simulink model "Citation_FlightGear_v2"  (R2026a)
settings: Solver=ode5  StopTime=10  FixedStep=0.01  EnableMultiTasking=on
InitFcn:
  | run('initcit.m')
  | run('id_init.m')
values from neighbouring files (symbols this model uses):
  beta_ref_max = 5*pi/180    (= 0.0872664625997)    [id_init.m]
  K_beta = 2    [id_init.m]
  K_da_to_p = p_ref_max/0.65    (= 0.537024385229)    [id_init.m]
  K_de_to_q = q_ref_max/0.35    (= 0.49866550057)    [id_init.m]
  K_dr_to_beta = beta_ref_max/0.38    (= 0.229648585789)    [id_init.m]
  Kaw_p = 1/Taw_p    (= 2)    [id_init.m]
  Kaw_q = 1/Taw_q    (= 2)    [id_init.m]
  Kaw_r = 1/Taw_r    (= 2)    [id_init.m]
  Ki_p = 5.0    (= 5)    [id_init.m]
  Ki_p_classical = -0.5    [id_init.m]
  Ki_q = 5.0    (= 5)    [id_init.m]
  Ki_q_classical = -0.1    [id_init.m]
  Ki_r = 5.0    (= 5)    [id_init.m]
  Ki_r_classical = -0.1    [id_init.m]
  Kp_p = 4.5    [id_init.m]
  Kp_p_classical = -1    [id_init.m]
  Kp_q = 4.5    [id_init.m]
  Kp_q_classical = -2    [id_init.m]
  Kp_r = 4.5    [id_init.m]
  Kp_r_classical = -2    [id_init.m]
  p_ref_max = 20*pi/180    (= 0.349065850399)    [id_init.m]
  PL0 = 10000*eye(6)    [id_init.m]
  PM0 = 10000*eye(4)    [id_init.m]
  PN0 = 10000*eye(6)    [id_init.m]
  PX0 = 10000*eye(5)    [id_init.m]
  PY0 = 10000*eye(6)    [id_init.m]
  PZ0 = 10000*eye(4)    [id_init.m]
  q_ref_max = 10*pi/180    (= 0.174532925199)    [id_init.m]
  r_ref_max = 10*pi/180    (= 0.174532925199)    [id_init.m]
  tau_cmd = 0.5    [id_init.m]
  thetaL0 = [       7.0957952465296537e-06 ... (first row only)    [id_init.m]
  thetaM0 = [       1.2280209971618383e-02 ... (first row only)    [id_init.m]
  thetaN0 = [      -4.9609095125384690e-06 ... (first row only)    [id_init.m]
  thetaX0 = zeros(5,1)    [id_init.m]
  thetaY0 = zeros(6,1)    [id_init.m]
  thetaZ0 = zeros(4,1)    [id_init.m]
  TL = 7.0875e-06    [id_init.m]
  TM = 3.2564e-06    [id_init.m]
  TN = 5.4692e-07    [id_init.m]
  TX = 2.2784e-06    [id_init.m]
  TY = 8.0633e-07    [id_init.m]
  TZ = 2.8004e-05    [id_init.m]
  Vw915 = 0    [initcit.m]
  winddir = -27*(pi/180)    (= -0.471238898038)    [initcit.m]
  x0 = []    [cessnac550_3d_sfnc.m]
undefined symbols (not defined in the file or in its folder): chord, cv1, cv2, cv3, cv4, deltagmax1, deltagmax2, deltagmax3, deltagmax4, Deng, ealphag, ealphas, g0, hDME, hGS, kt1, kt2, kt3, lh, massinit, matbuaf, matdaf, matdam, matdbbf, matdeaf, matdgaf, matdqaf, matduaf, matdwaw, matedhr, mateif, matelhr, matemhr, matemv1, matemv2, matemve, matetam, mateuaf, matfaaf, matfaxl, matff, matibaf, matibb, matibmh, matipaf, matipmh, matiraf, matiuaf, matiwaf, matlaf, matlam, matleaf, matleam, matlgaf, matlqaf, matluaf, matmaaf, matmaam, matmaf, matmam ... (+78)
libraries: simulink x13, aerolibfltsims x3, aerolibconvert2 x2, aerolibobsolete x1, aerolibanimutils x1
(part 1 of 5)
settings Model: ExtModeTrigMode=oneshot  ExtModeArmWhenConnect=off  Creator=laurensvaneykeren  LastModifiedBy=eltjo
settings DataIOCC: SignalLoggingSaveFormat=ModelDataLogs  SignalLoggingName=sigsOut
settings OptimizationCC: BooleanDataType=off
settings DebuggingCC: SaveWithParameterizedLinksMsg=none  UnderspecifiedInitializationDetection=Classic  SignalResolutionControl=TryResolveAllWithWarning  MultiTaskDSMMsg=warning  MultiTaskCondExecSysMsg=none
settings HardwareCC: ProdHWDeviceType=32-bit Generic  TargetUnknown=on
settings RTWCC: SystemTargetFile=grt_malloc.tlc  GenCodeOnly=on  TemplateMakefile=grt_malloc_default_tmf
settings GRTTargetCC: UseMalloc=on  CombineOutputUpdateFcns=off  GRTInterface=on

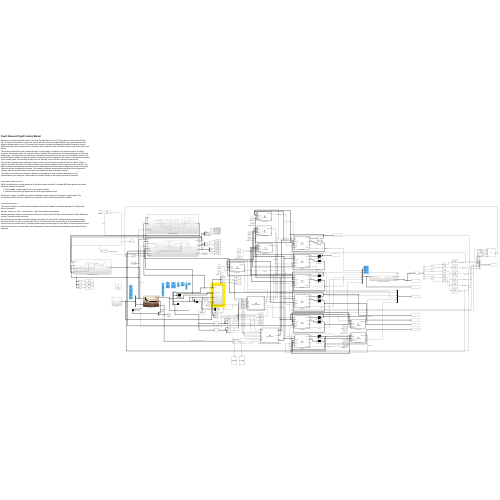
[thumbnail: Simulink's stored preview of the top-level diagram]
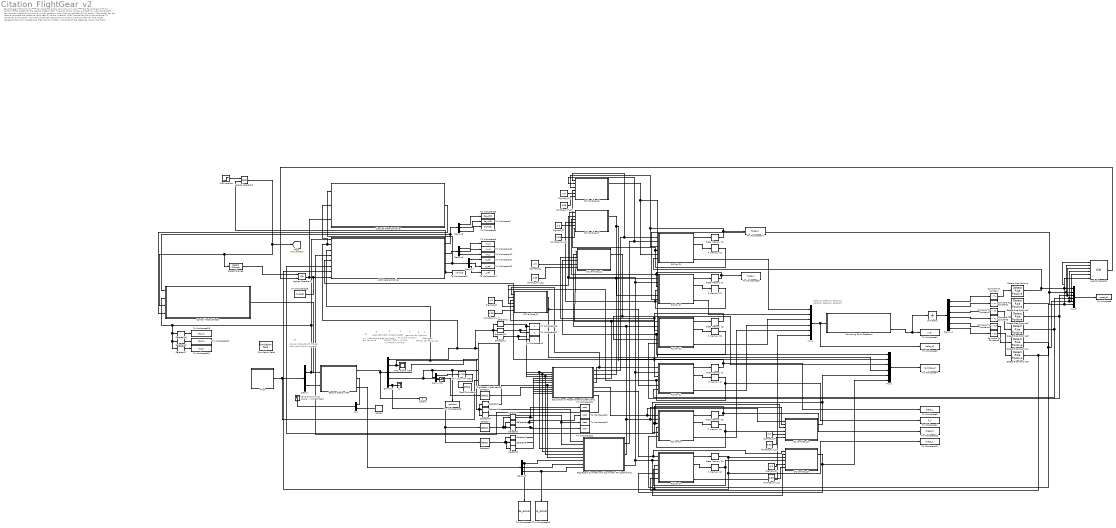
== system Citation_FlightGear_v2 ==
  note: Fault-Tolerant Flight Control Model
      | Welcome to the main Simulink model of the Fault-Tolerant Flight Control (FTFC) system for the Cessna Citation 500. The goal of this model is to test how well the aircraft can maintain stable flight during normal operation and when an actuator failure occurs. The model can be used to compare the Adaptive Nonlinear Dynamic Inversion (ANDI) controller with a conventional PI controller, and to study how both controllers respond to an aileron hard-over failure.
      | The model represents the main closed-loop flight control system. It consists of the reference inputs, the flight controller, the actuator model, the nonlinear Cessna Citation 500 aircraft model, the feedback signals, and the fault-related logic. The reference inputs specify the desired aircraft response and are sent to the selected controller. The controller then calculates the required actuator commands, which are passed to the actuator subsystem and applied to the aircraft model. The resulting aircraft motion is fed back to the controller, closing the control loop.
      | The actuator subsystem also contains the failure model used to introduce the aileron hard-over failure. When a failure is activated, the effect of the failed actuator can be studied together with the response of the controller. The ANDI controller uses feedback information and the estimated control effectiveness to adjust the control commands when the actuator configuration changes. This makes it possible to compare the nominal and failure cases and evaluate how well the fault-tolerant controller can maintain the desired aircraft behaviour.
      | The model can therefore be operated in different configurations to study controller performance, fault accommodation and tolerance, and the effect of actuator failures on the closed-loop aircraft dynamics.
      |
      | Switching Between ANDI and PI Control
      | ANDI is enabled during normal operation of the fault-tolerant controller. To disable ANDI and operate the aircraft using the classical PI controller:
      | Set the ANDI enable signal to 0 for the entire simulation.
      | Disconnect the valid_B signal from the AND logical operator block.
      | With these changes, the ANDI control path is disabled and the classical PI controller is used instead. This configuration can be used as a baseline for comparison with the fault-tolerant ANDI controller.
      |
      | Activating the Actuator Failure
      | The model contains an actuator failure mechanism that can be enabled or disabled manually. To configure the failure, navigate to:
      | Cessna Citation 500 → Actuators → Failure Mode Activation
      | Enabling Failure Mode Activation introduces an aileron hard-over failure into the aircraft model. Disabling it restores nominal actuator behaviour.
      | By combining the controller and failure settings, the model can be used to investigate several important cases, including nominal PI control, nominal ANDI control, PI control during an actuator failure, and fault-tolerant ANDI control during an actuator failure. Comparing these cases provides insight into the ability of the fault-tolerant control architecture to detect, accommodate, and compensate for actuator failures while maintaining the desired aircraft response.
  note: de
      | da
      | dr
      | dte
      | dta
      | dtr
      | df
      | gear
      | pla1
      | pla2
      | turb 8x
      | terr elev
  note: p
      | q
      | r
      | vtas
      | alpha
      | beta
      | phi
      | theta
      | psi
      | he
      | xe
      | ye
  note: pdot
      | qdot
      | rdot
      | VTASdot
      | hedot
  note: hradio
      | Mach
      | u_wind_e
      | v_wind_e
      | w_wind_e
  note: anxb
      | anyb
      | anzb
      | n
  note: gamma
      | chi
      | Vground
  note: flaps
      | gear
  note: FFl
      | N1l
      | N2l
      | FFr
      | N1r
      | N2r
  note: 12
  note: 5
  note: 5
  note: 4
  note: 3
  note: 6
  note: 2
  note: 19
  note: delta_CX
      | delta_CY
      | delta_CZ
      | delta_Cl
      | delta_Cm
      | delta_Cn
  2 : Terminator
  3 : Terminator
  ANDI Rate Controller : Subsystem
  ANDI enable : Step  Time=0  InitialValue=1  SampleTime=0
  Alt < 10 m => Stop : Fcn  Expr=u<10
  CIC lambda_CX : MATLAB Function  TreatAsAtomicUnit=on
  CIC lambda_CY : MATLAB Function  TreatAsAtomicUnit=on
  CIC lambda_CZ : MATLAB Function  TreatAsAtomicUnit=on
  CIC lambda_Cl : MATLAB Function  TreatAsAtomicUnit=on
  CIC lambda_Cm : MATLAB Function  TreatAsAtomicUnit=on
  CIC lambda_Cn : MATLAB Function  TreatAsAtomicUnit=on
  Calculation of Force/Moments Coefficients : MATLAB Function  TreatAsAtomicUnit=on
  Cessna Citation 500 : Subsystem  mask(Citation Aircraft Model){trimdatafile=}
      mask prompts: trimdatafile "Trim Condition"
      mask init:
      | initcit;
      mask Display:
      | image(imread('Citation.jpg'))
      | port_label('input', 1, 'Inputs')
      | port_label('input', 2, 'Environment')
      | port_label('output', 1, 'Outputs')
      | port_label('output', 2, 'Trim inputs')
  Classical Rate Controller : Subsystem
  Compare To Constant : simulink/Logic and Bit Operations/Compare To Constant  relop=>  const=TX  OutDataTypeStr=boolean
  Compare To Constant1 : simulink/Logic and Bit Operations/Compare To Constant  relop=>  const=TY  OutDataTypeStr=boolean
  Compare To Constant2 : simulink/Logic and Bit Operations/Compare To Constant  relop=>  const=TZ  OutDataTypeStr=boolean
  Compare To Constant3 : simulink/Logic and Bit Operations/Compare To Constant  relop=>  const=TL  OutDataTypeStr=boolean
  Compare To Constant4 : simulink/Logic and Bit Operations/Compare To Constant  relop=>  const=TM  OutDataTypeStr=boolean
  Compare To Constant5 : simulink/Logic and Bit Operations/Compare To Constant  relop=>  const=TN  OutDataTypeStr=boolean
  Control Mode Selector : Subsystem
  Demux : Demux  Outputs=[10 9]
      settings: DisplayOption=none
  Demux1 : Demux  Outputs=[3 3 3 3 25]
      settings: DisplayOption=none
  Demux2 : Demux  Outputs=[1 2]
  Demux{3,5..7} (4 alike) : Demux  Outputs=3
  Demux4 : Demux  Outputs=6
  Detect Change : simulink/Logic and Bit Operations/Detect Change  vinit=0  OutDataTypeStr=boolean
  Detect Rise Positive{,1..5} (6 alike) : simulink/Logic and Bit Operations/Detect Rise Positive  vinit=0  OutDataTypeStr=boolean
  FlightGear Visualisation : Subsystem
  Logical Operator : Logic  Operator=OR  Inputs=6  AllPortsSameDT=off  OutDataTypeStr=boolean
  Logical Operator1 : Logic  Operator=OR  AllPortsSameDT=off  OutDataTypeStr=boolean
  Logical Operator2 : Logic  AllPortsSameDT=off  OutDataTypeStr=boolean
  Monitoring Fault Detection : Subsystem
  Mux : Mux  Inputs=2
  Mux1 : Mux  Inputs=6
  Mux2 : Mux  Inputs=6
  Mux3 : Mux  Inputs=6
  P memory CX : Memory  InitialCondition=PX0
  P memory CY : Memory  InitialCondition=PY0
  P memory CZ : Memory  InitialCondition=PZ0
  P memory Cl : Memory  InitialCondition=PL0
  P memory Cm : Memory  InitialCondition=PM0
  P memory Cn : Memory  InitialCondition=PN0
  Pilot : Subsystem
  RLS for CL : MATLAB Function  TreatAsAtomicUnit=on
  RLS for CX : MATLAB Function  TreatAsAtomicUnit=on
  RLS for CY : MATLAB Function  TreatAsAtomicUnit=on
  RLS for CZ : MATLAB Function  TreatAsAtomicUnit=on
  RLS for Cm : MATLAB Function  TreatAsAtomicUnit=on
  RLS for Cn : MATLAB Function  TreatAsAtomicUnit=on
  Regressors Symmetr. and Asymmetr. F/M Coefficients : MATLAB Function  TreatAsAtomicUnit=on
  Selector : Selector  InputPortWidth=25  IndexOptions=Index vector (dialog)  Indices=[1 2 3]  OutputSizes=1
  Selector1 : Selector  InputPortWidth=3  IndexOptions=Index vector (dialog)  Indices=1  OutputSizes=1
  Selector{5,8,10,13} (4 alike) : Selector  InputPortWidth=3  IndexOptions=Index vector (dialog)  Indices=[2]  OutputSizes=1
  Selector{6,9,11,14} (4 alike) : Selector  InputPortWidth=3  IndexOptions=Index vector (dialog)  Indices=[3]  OutputSizes=1
  Selector{3..4,7,12} (4 alike) : Selector  InputPortWidth=3  IndexOptions=Index vector (dialog)  Indices=[1]  OutputSizes=1
  Selector15 : Selector  InputPortWidth=10  IndexOptions=Index vector (dialog)  Indices=[1]  OutputSizes=1
  Selector16 : Selector  InputPortWidth=10  IndexOptions=Index vector (dialog)  Indices=[2]  OutputSizes=1
  Selector17 : Selector  InputPortWidth=10  IndexOptions=Index vector (dialog)  Indices=[3]  OutputSizes=1
  Selector2 : Selector  InputPortWidth=25  IndexOptions=Index vector (dialog)  Indices=[11 12 13]  OutputSizes=1
  Sigma0_CX : Constant  Value=0.5
  Sigma0_CY : Constant  Value=0.5
  Sigma0_CZ : Constant  Value=0.5
  Sigma0_Cl : Constant  Value=0.5
  Sigma0_Cm : Constant  Value=0.5
  Sigma0_Cn : Constant  Value=0.5
  Simulation Pace : aerolibanimutils/Simulation Pace  SimulationPace=1  SleepMode=MATLAB Thread  OutputPaceError=off  SampleTime=-1
      settings: AttributesFormatString=%<SimulationPace> sec/sec
  Stop Simulation : Stop
  To Workspace : ToWorkspace  VariableName=reset_all  SaveFormat=Timeseries  SampleTime=-1
  To Workspace1 : ToWorkspace  VariableName=P_L  SaveFormat=Timeseries  SampleTime=-1
  To Workspace10 : ToWorkspace  VariableName=nu_q  SaveFormat=Timeseries  SampleTime=-1
  To Workspace11 : ToWorkspace  VariableName=p_ref  SaveFormat=Timeseries  SampleTime=-1
  To Workspace12 : ToWorkspace  VariableName=nu_r  SaveFormat=Timeseries  SampleTime=-1
  To Workspace13 : ToWorkspace  VariableName=q_ref  SaveFormat=Timeseries  SampleTime=-1
  To Workspace14 : ToWorkspace  VariableName=r_ref  SaveFormat=Timeseries  SampleTime=-1
  To Workspace15 : ToWorkspace  VariableName=valid_B  SaveFormat=Timeseries  SampleTime=-1
  To Workspace16 : ToWorkspace  VariableName=p  SaveFormat=Timeseries  SampleTime=-1
  To Workspace17 : ToWorkspace  VariableName=q  SaveFormat=Timeseries  SampleTime=-1
  To Workspace18 : ToWorkspace  VariableName=r  SaveFormat=Timeseries  SampleTime=-1
  To Workspace19 : ToWorkspace  VariableName=beta  SaveFormat=Timeseries  SampleTime=-1
  To Workspace2 : ToWorkspace  VariableName=Jvar  SaveFormat=Timeseries  SampleTime=-1
  To Workspace20 : ToWorkspace  VariableName=qdot  SaveFormat=Timeseries  SampleTime=-1
  To Workspace21 : ToWorkspace  VariableName=pdot  SaveFormat=Timeseries  SampleTime=-1
  To Workspace22 : ToWorkspace  VariableName=rdot  SaveFormat=Timeseries  SampleTime=-1
  To Workspace23 : ToWorkspace  VariableName=theta_M  SaveFormat=Timeseries  SampleTime=-1
  To Workspace24 : ToWorkspace  VariableName=theta_N  SaveFormat=Timeseries  SampleTime=-1
  To Workspace25 : ToWorkspace  VariableName=PI_reset  SaveFormat=Timeseries  SampleTime=-1
  To Workspace26 : ToWorkspace  VariableName=theta_Y  SaveFormat=Timeseries  SampleTime=-1
  To Workspace27 : ToWorkspace  VariableName=theta_X  SaveFormat=Timeseries  SampleTime=-1
  To Workspace28 : ToWorkspace  VariableName=position  SaveFormat=Timeseries  SampleTime=-1
  To Workspace29 : ToWorkspace  VariableName=de_joy  SaveFormat=Timeseries  SampleTime=-1
  To Workspace3 : ToWorkspace  VariableName=delta_all  SaveFormat=Timeseries  SampleTime=-1
  To Workspace30 : ToWorkspace  VariableName=da_joy  SaveFormat=Timeseries  SampleTime=-1
  To Workspace31 : ToWorkspace  VariableName=dr_joy  SaveFormat=Timeseries  SampleTime=-1
  To Workspace32 : ToWorkspace  VariableName=de_actual  SaveFormat=Timeseries  SampleTime=-1
  To Workspace33 : ToWorkspace  VariableName=dr_actual  SaveFormat=Timeseries  SampleTime=-1
  To Workspace4 : ToWorkspace  VariableName=lambda_all  SaveFormat=Timeseries  SampleTime=-1
  To Workspace5 : ToWorkspace  VariableName=de_ANDI  SaveFormat=Timeseries  SampleTime=-1
  To Workspace6 : ToWorkspace  VariableName=dr_ANDI  SaveFormat=Timeseries  SampleTime=-1
  To Workspace7 : ToWorkspace  VariableName=da_ANDI  SaveFormat=Timeseries  SampleTime=-1
  To Workspace8 : ToWorkspace  VariableName=theta_L  SaveFormat=Timeseries  SampleTime=-1
  To Workspace9 : ToWorkspace  VariableName=nu_p  SaveFormat=Timeseries  SampleTime=-1
  Unit Delay : UnitDelay  SampleTime=0.01
  Using this as input would result in trimmed flight : Terminator
  "VTAS, alpha, beta" : Scope
      settings: ActiveDisplayYMinimum=-192.0765592563377  ActiveDisplayYMaximum=190.51852643229006  DataLoggingVariableName=ScopeData7
  lambda_min_CX : Constant  Value=0.95
  lambda_min_CY : Constant  Value=0.95
  lambda_min_CZ : Constant  Value=0.95
  lambda_min_Cl : Constant  Value=0.95
  lambda_min_Cm : Constant  Value=0.95
  lambda_min_Cn : Constant  Value=0.95
  theta Memory CX : Memory  InitialCondition=thetaX0
  theta Memory CY : Memory  InitialCondition=thetaY0
  theta Memory CZ : Memory  InitialCondition=thetaZ0
  theta Memory Cl : Memory  InitialCondition=thetaL0
  theta Memory Cm : Memory  InitialCondition=thetaM0
  theta Memory Cn : Memory  InitialCondition=thetaN0
  zeroes : Constant  Value=[0 0 0 0 0 0 0 0 0]
  Output : Outport
  tag scope: ANDI_ENABLE=global
  wires:
  Demux/1 -> Selector17/1, Selector16/1, Selector15/1, Control Mode Selector/2(pilot_u), ANDI Rate Controller/1(pilot_u)
  Cessna Citation 500/1(output) -> Demux1/1, Output/1
  Demux/2 -> Cessna Citation 500/2(Environment)
  Cessna Citation 500/2(Trimmed input) -> Mux/1  "Input values in trim condition"
  zeroes/1 -> Mux/2
  Mux/1 -> Using this as input would result in trimmed flight/1
  Demux1/1 -> Classical Rate Controller/2(pqr), ANDI Rate Controller/2(pqr), Selector11/1, Selector12/1, Selector10/1, FlightGear Visualisation/1("[p,q,r]")  "p,q,r"
  Demux1/2 -> ANDI Rate Controller/3("VTAS, alpha, beta"), Selector14/1, Selector3/1, Selector13/1, "VTAS, alpha, beta"/1
  Alt < 10 m => Stop/1 -> Stop Simulation/1
  Demux1/5 -> Selector2/1, Selector/1, 2/1
  Demux1/4 -> Selector1/1, Demux2/1, To Workspace28/1, FlightGear Visualisation/3("[he, xe, ye]")
  Demux2/1 -> Alt < 10 m => Stop/1
  Pilot/1(Input) -> FlightGear Visualisation/4(u), Demux/1
  Demux2/2 -> 3/1
  Demux1/3 -> FlightGear Visualisation/2(" [phi, theta, psi]")  "phi,theta,psi"
  Cessna Citation 500/3(Outport SysID Deflections) -> Demux3/1  "de_healthy, da_healthy, dr_healthy"
  Selector1/1 -> Calculation of Force/Moments Coefficients/8(h)  "he"
  Selector3/1 -> Regressors Symmetr. and Asymmetr. F/M Coefficients/6(V), Calculation of Force/Moments Coefficients/7(V)  "VTAS"
  Selector/1 -> Selector4/1, Selector5/1, Selector6/1
  Selector4/1 -> To Workspace21/1, Calculation of Force/Moments Coefficients/4(pdot)  "pdot"
  Selector5/1 -> To Workspace20/1, Calculation of Force/Moments Coefficients/5(qdot)  "qdot"
  Selector6/1 -> To Workspace22/1, Calculation of Force/Moments Coefficients/6(rdot)  "rdot"
  Selector7/1 -> Calculation of Force/Moments Coefficients/9(anxb)  "anxb"
  Selector9/1 -> Calculation of Force/Moments Coefficients/11(anzb)  "anzb"
  Selector8/1 -> Calculation of Force/Moments Coefficients/10(anyb)  "anyb"
  Selector2/1 -> Selector9/1, Selector8/1, Selector7/1
  Selector12/1 -> To Workspace16/1, Regressors Symmetr. and Asymmetr. F/M Coefficients/3(p), Calculation of Force/Moments Coefficients/1(p)  "p"
  Selector10/1 -> To Workspace17/1, Regressors Symmetr. and Asymmetr. F/M Coefficients/4(q), Calculation of Force/Moments Coefficients/2(q)  "q"
  Selector11/1 -> To Workspace18/1, Regressors Symmetr. and Asymmetr. F/M Coefficients/5(r), Calculation of Force/Moments Coefficients/3(r)  "r"
  Selector13/1 -> Regressors Symmetr. and Asymmetr. F/M Coefficients/1(alpha)  "alpha"
  Selector14/1 -> Regressors Symmetr. and Asymmetr. F/M Coefficients/2(beta), To Workspace19/1  "beta"
  Demux3/1 -> Regressors Symmetr. and Asymmetr. F/M Coefficients/7(de), To Workspace32/1  "de_healthy"
  Demux3/2 -> Regressors Symmetr. and Asymmetr. F/M Coefficients/8(da)  "da_healthy"
  Demux3/3 -> Regressors Symmetr. and Asymmetr. F/M Coefficients/9(dr), To Workspace33/1  "dr_healthy"
  Regressors Symmetr. and Asymmetr. F/M Coefficients/3(phiLat) -> CIC lambda_Cn/2(phi), RLS for Cn/2(phi), RLS for CL/2(phi), RLS for CY/2(phi), CIC lambda_Cl/2(phi), CIC lambda_CY/2(phi)
  RLS for Cn/1(theta_new) -> theta Memory Cn/1
  theta Memory Cn/1 -> To Workspace24/1, ANDI Rate Controller/7(thetaN), RLS for Cn/3(theta_old), CIC lambda_Cn/3(theta_old)
  RLS for Cn/2(P_new) -> P memory Cn/1
  P memory Cn/1 -> RLS for Cn/4(P_old), CIC lambda_Cn/4(P_old)
  Calculation of Force/Moments Coefficients/1(CX) -> CIC lambda_CX/1(z), RLS for CX/1(z)
  P memory CX/1 -> CIC lambda_CX/4(P_old), RLS for CX/4(P_old)
  theta Memory CX/1 -> CIC lambda_CX/3(theta_old), RLS for CX/3(theta_old), To Workspace27/1
  RLS for CX/2(P_new) -> P memory CX/1
  RLS for CX/1(theta_new) -> theta Memory CX/1
  Regressors Symmetr. and Asymmetr. F/M Coefficients/1(phiX) -> CIC lambda_CX/2(phi), RLS for CX/2(phi)
  P memory CY/1 -> CIC lambda_CY/4(P_old), RLS for CY/4(P_old)
  theta Memory CY/1 -> CIC lambda_CY/3(theta_old), RLS for CY/3(theta_old), To Workspace26/1
  RLS for CY/2(P_new) -> P memory CY/1
  RLS for CY/1(theta_new) -> theta Memory CY/1
  Calculation of Force/Moments Coefficients/2(CY) -> RLS for CY/1(z), CIC lambda_CY/1(z)
  P memory CZ/1 -> RLS for CZ/4(P_old), CIC lambda_CZ/4(P_old)
  theta Memory CZ/1 -> CIC lambda_CZ/3(theta_old), RLS for CZ/3(theta_old)
  CIC lambda_CZ/1(lambda_ad) -> RLS for CZ/5(lambda), Mux2/3  "lambda_CZ"
  RLS for CZ/2(P_new) -> P memory CZ/1
  RLS for CZ/1(theta_new) -> theta Memory CZ/1
  Calculation of Force/Moments Coefficients/3(CZ) -> RLS for CZ/1(z), CIC lambda_CZ/1(z)
  Regressors Symmetr. and Asymmetr. F/M Coefficients/2(phiZM) -> CIC lambda_Cm/2(phi), RLS for Cm/2(phi), RLS for CZ/2(phi), CIC lambda_CZ/2(phi)
  P memory Cl/1 -> To Workspace1/1, CIC lambda_Cl/4(P_old), RLS for CL/4(P_old)
  theta Memory Cl/1 -> To Workspace8/1, ANDI Rate Controller/5(thetaL), RLS for CL/3(theta_old), CIC lambda_Cl/3(theta_old)
  CIC lambda_Cl/1(lambda_ad) -> Mux2/4, RLS for CL/5(lambda)  "lambda_Cl"
  RLS for CL/2(P_new) -> P memory Cl/1
  RLS for CL/1(theta_new) -> theta Memory Cl/1
  P memory Cm/1 -> RLS for Cm/4(P_old), CIC lambda_Cm/4(P_old)
  theta Memory Cm/1 -> To Workspace23/1, ANDI Rate Controller/6(thetaM), CIC lambda_Cm/3(theta_old), RLS for Cm/3(theta_old)
  RLS for Cm/2(P_new) -> P memory Cm/1
  RLS for Cm/1(theta_new) -> theta Memory Cm/1
  Calculation of Force/Moments Coefficients/4(Cl) -> CIC lambda_Cl/1(z), RLS for CL/1(z)
  Calculation of Force/Moments Coefficients/5(Cm) -> CIC lambda_Cm/1(z), RLS for Cm/1(z)
  Calculation of Force/Moments Coefficients/6(Cn) -> CIC lambda_Cn/1(z), RLS for Cn/1(z)
  RLS for CX/4(innovation) -> Mux1/1  "delta_CX"
  RLS for CY/4(innovation) -> Mux1/2  "delta_CY"
  RLS for CZ/4(innovation) -> Mux1/3  "delta_CZ"
  RLS for CL/4(innovation) -> Mux1/4  "delta_Cl"
  RLS for Cm/4(innovation) -> Mux1/5  "delta_Cm"
  RLS for Cn/4(innovation) -> Mux1/6  "delta_Cn"
  Mux1/1 -> To Workspace3/1, Monitoring Fault Detection/1(innovations)
  Sigma0_CX/1 -> CIC lambda_CX/5(Sigma0)
  lambda_min_CX/1 -> CIC lambda_CX/6(lambda_min)
  CIC lambda_CX/1(lambda_ad) -> Mux2/1, RLS for CX/5(lambda)  "lambda_CX"
  Sigma0_CY/1 -> CIC lambda_CY/5(Sigma0)
  lambda_min_CY/1 -> CIC lambda_CY/6(lambda_min)
  CIC lambda_CY/1(lambda_ad) -> Mux2/2, RLS for CY/5(lambda)  "lambda_CY"
  Sigma0_CZ/1 -> CIC lambda_CZ/5(Sigma0)
  lambda_min_CZ/1 -> CIC lambda_CZ/6(lambda_min)
  Sigma0_Cl/1 -> CIC lambda_Cl/5(Sigma0)
  lambda_min_Cl/1 -> CIC lambda_Cl/6(lambda_min)
  Sigma0_Cm/1 -> CIC lambda_Cm/5(Sigma0)
  lambda_min_Cm/1 -> CIC lambda_Cm/6(lambda_min)
  CIC lambda_Cm/1(lambda_ad) -> Mux2/5, RLS for Cm/5(lambda)  "lambda_Cm"
  Sigma0_Cn/1 -> CIC lambda_Cn/5(Sigma0)
  lambda_min_Cn/1 -> CIC lambda_Cn/6(lambda_min)
  CIC lambda_Cn/1(lambda_ad) -> Mux2/6, RLS for Cn/5(lambda)  "lambda_Cn"
  Monitoring Fault Detection/3(VARIANCE) -> Unit Delay/1, To Workspace2/1  "Variance"
  Mux2/1 -> To Workspace4/1
  Demux4/1 -> Compare To Constant/1  "Jvar_X"
  Demux4/2 -> Compare To Constant1/1  "Jvar_Y"
  Demux4/3 -> Compare To Constant2/1  "Jvar_Z"
  Demux4/4 -> Compare To Constant3/1  "Jvar_L"
  Demux4/5 -> Compare To Constant4/1  "Jvar_M"
  Demux4/6 -> Compare To Constant5/1  "Jvar_N"
  Compare To Constant/1 -> Detect Rise Positive/1
  Compare To Constant1/1 -> Detect Rise Positive1/1
  Compare To Constant2/1 -> Detect Rise Positive2/1
  Compare To Constant3/1 -> Detect Rise Positive3/1
  Compare To Constant5/1 -> Detect Rise Positive5/1
  Compare To Constant4/1 -> Detect Rise Positive4/1
  Detect Rise Positive/1 -> RLS for CX/6(reset), Logical Operator/1, Mux3/1  "reset_CX"
  Detect Rise Positive1/1 -> Logical Operator/2, Mux3/2, RLS for CY/6(reset)  "reset_CY"
  Detect Rise Positive2/1 -> RLS for CZ/6(reset), Logical Operator/3, Mux3/3  "reset_CZ"
  Detect Rise Positive3/1 -> RLS for CL/6(reset), Logical Operator/4, Mux3/4  "reset_CL"
  Detect Rise Positive4/1 -> Logical Operator/5, Mux3/5, RLS for Cm/6(reset)  "reset_CM"
  Detect Rise Positive5/1 -> RLS for Cn/6(reset), Mux3/6, Logical Operator/6  "reset_CN"
  Mux3/1 -> To Workspace/1
  Unit Delay/1 -> Demux4/1
  Calculation of Force/Moments Coefficients/7(rho) -> ANDI Rate Controller/4(rho)
  ANDI enable/1 -> Logical Operator2/1
  ANDI Rate Controller/1(u_ANDI) -> Demux5/1, Control Mode Selector/1(u_ANDI)
  Control Mode Selector/1(aircraft_u) -> Cessna Citation 500/1(Inputs)  "aircraft_u"
  Logical Operator/1 -> Logical Operator1/2  "model_reset"
  Detect Change/1 -> Logical Operator1/1  "mode_change"
  Logical Operator1/1 -> Classical Rate Controller/3(PI_reset), To Workspace25/1, ANDI Rate Controller/8(PI_reset)  "PI_reset"
  Demux5/1 -> To Workspace5/1  "de_ANDI"
  Demux5/2 -> To Workspace7/1  "da_ANDI"
  Demux5/3 -> To Workspace6/1  "dr_ANDI"
  ANDI Rate Controller/2(nu) -> Demux6/1
  Demux6/1 -> To Workspace9/1  "nu_p"
  Demux6/2 -> To Workspace10/1  "nu_q"
  Demux6/3 -> To Workspace12/1  "nu_r"
  ANDI Rate Controller/3(refs) -> Classical Rate Controller/1(refs), Demux7/1
  Demux7/1 -> To Workspace11/1  "p_ref"
  Demux7/2 -> To Workspace13/1  "q_ref"
  Demux7/3 -> To Workspace14/1  "r_ref"
  ANDI Rate Controller/4(valid_B) -> To Workspace15/1, Logical Operator2/2  "valid_B"
  Classical Rate Controller/1(u_classical) -> Control Mode Selector/4(u_classical)
  Selector15/1 -> To Workspace29/1
  Selector16/1 -> To Workspace30/1
  Selector17/1 -> To Workspace31/1
  Logical Operator2/1 -> Detect Change/1, Control Mode Selector/3(ANDI_enable), [ANDI_ENABLE]

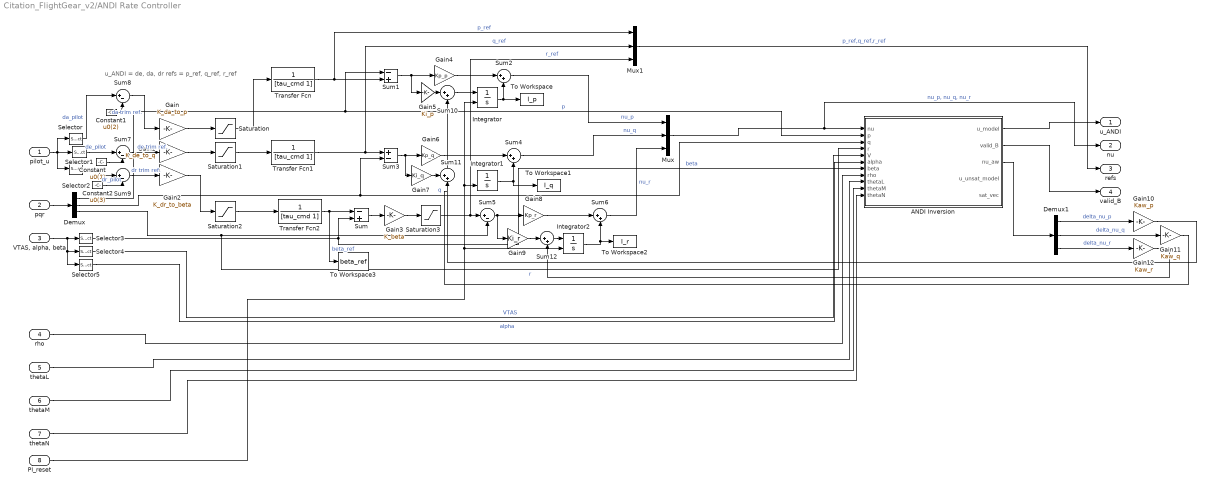
== system Citation_FlightGear_v2/ANDI Rate Controller ==
  note: u_ANDI = de, da, dr
      | refs = p_ref, q_ref, r_ref
  pilot_u : Inport
  pqr : Inport  Port=2
  "VTAS, alpha, beta" : Inport  Port=3
  rho : Inport  Port=4
  thetaL : Inport  Port=5
  thetaM : Inport  Port=6
  thetaN : Inport  Port=7
  PI_reset : Inport  Port=8
  ANDI Inversion : MATLAB Function  TreatAsAtomicUnit=on
  Constant : Constant  Value=u0(1)
  Constant1 : Constant  Value=u0(2)
  Constant2 : Constant  Value=u0(3)
  Demux : Demux  Outputs=3
  Demux1 : Demux  Outputs=3
  Gain : Gain  Gain=K_da_to_p
  Gain1 : Gain  Gain=K_de_to_q
  Gain10 : Gain  Gain=Kaw_p
  Gain11 : Gain  Gain=Kaw_q
  Gain12 : Gain  Gain=Kaw_r
  Gain2 : Gain  Gain=K_dr_to_beta
  Gain3 : Gain  Gain=K_beta
  Gain4 : Gain  Gain=Kp_p
  Gain5 : Gain  Gain=Ki_p
  Gain6 : Gain  Gain=Kp_q
  Gain7 : Gain  Gain=Ki_q
  Gain8 : Gain  Gain=Kp_r
  Gain9 : Gain  Gain=Ki_r
  Integrator : Integrator  ExternalReset=rising
  Integrator1 : Integrator  ExternalReset=rising
  Integrator2 : Integrator  ExternalReset=rising
  Mux : Mux  Inputs=3
  Mux1 : Mux  Inputs=3
  Saturation : Saturate  UpperLimit=p_ref_max  LowerLimit=-p_ref_max
  Saturation1 : Saturate  UpperLimit=q_ref_max  LowerLimit=-q_ref_max
  Saturation2 : Saturate  UpperLimit=beta_ref_max  LowerLimit=-beta_ref_max
  Saturation3 : Saturate  UpperLimit=r_ref_max  LowerLimit=-r_ref_max
  Selector : Selector  InputPortWidth=10  IndexOptions=Index vector (dialog)  Indices=[2]  OutputSizes=1
  Selector1 : Selector  InputPortWidth=10  IndexOptions=Index vector (dialog)  Indices=[1]  OutputSizes=1
  Selector2 : Selector  InputPortWidth=10  IndexOptions=Index vector (dialog)  Indices=[3]  OutputSizes=1
  Selector3 : Selector  InputPortWidth=3  IndexOptions=Index vector (dialog)  Indices=[3]  OutputSizes=1
  Selector4 : Selector  InputPortWidth=3  IndexOptions=Index vector (dialog)  Indices=[1]  OutputSizes=1
  Selector5 : Selector  InputPortWidth=3  IndexOptions=Index vector (dialog)  Indices=[2]  OutputSizes=1
  Sum : Sum  Inputs=-+
  Sum1 : Sum  Inputs=-+
  Sum{2,4,6,10..12} (6 alike) : Sum  Inputs=|++
  Sum3 : Sum  Inputs=+-
  Sum{5,7..9} (4 alike) : Sum  Inputs=|+-
  To Workspace : ToWorkspace  VariableName=I_p  SaveFormat=Timeseries  SampleTime=-1
  To Workspace1 : ToWorkspace  VariableName=I_q  SaveFormat=Timeseries  SampleTime=-1
  To Workspace2 : ToWorkspace  VariableName=I_r  SaveFormat=Timeseries  SampleTime=-1
  To Workspace3 : ToWorkspace  VariableName=beta_ref  SaveFormat=Timeseries  SampleTime=-1
  Transfer Fcn : TransferFcn  Denominator=[tau_cmd 1]
  Transfer Fcn1 : TransferFcn  Denominator=[tau_cmd 1]
  Transfer Fcn2 : TransferFcn  Denominator=[tau_cmd 1]
  u_ANDI : Outport
  nu : Outport  Port=2
  refs : Outport  Port=3
  valid_B : Outport  Port=4
  wires:
  pilot_u/1 -> Selector2/1, Selector1/1, Selector/1
  Selector/1 -> Sum8/1  "da_pilot"
  Selector1/1 -> Sum7/1  "de_pilot"
  Selector2/1 -> Sum9/1  "dr_pilot"
  Gain/1 -> Saturation/1
  Saturation/1 -> Transfer Fcn/1
  Transfer Fcn/1 -> Sum1/2, Mux1/1  "p_ref"
  Gain1/1 -> Saturation1/1
  Saturation1/1 -> Transfer Fcn1/1
  Transfer Fcn1/1 -> Mux1/2, Sum3/1  "q_ref"
  Gain2/1 -> Saturation2/1
  Saturation2/1 -> Transfer Fcn2/1
  Transfer Fcn2/1 -> To Workspace3/1, Sum/1  "beta_ref"
  "VTAS, alpha, beta"/1 -> Selector5/1, Selector4/1, Selector3/1
  Selector3/1 -> ANDI Inversion/7(beta), Sum/2  "beta"
  Sum/1 -> Gain3/1
  Gain3/1 -> Saturation3/1
  Saturation3/1 -> Mux1/3, Sum5/1  "r_ref"
  pqr/1 -> Demux/1
  Demux/1 -> ANDI Inversion/2(p), Sum1/1  "p"
  Demux/2 -> Sum3/2, ANDI Inversion/3(q)  "q"
  Demux/3 -> ANDI Inversion/4(r), Sum5/2  "r"
  Sum1/1 -> Gain4/1, Gain5/1
  PI_reset/1 -> Integrator2/2, Integrator/2, Integrator1/2
  Integrator/1 -> Sum2/2, To Workspace/1
  Gain4/1 -> Sum2/1
  Sum2/1 -> Mux/1  "nu_p"
  Sum3/1 -> Gain7/1, Gain6/1
  Gain7/1 -> Sum11/1
  Gain6/1 -> Sum4/1
  Integrator1/1 -> Sum4/2, To Workspace1/1
  Sum4/1 -> Mux/2  "nu_q"
  Sum5/1 -> Gain8/1, Gain9/1
  Gain8/1 -> Sum6/1
  Gain9/1 -> Sum12/1
  Integrator2/1 -> Sum6/2, To Workspace2/1
  Sum6/1 -> Mux/3  "nu_r"
  Mux/1 -> nu/1, ANDI Inversion/1(nu)  "nu_p, nu_q, nu_r"
  Selector4/1 -> ANDI Inversion/5(V)  "VTAS"
  Selector5/1 -> ANDI Inversion/6(alpha)  "alpha"
  rho/1 -> ANDI Inversion/8(rho)
  thetaL/1 -> ANDI Inversion/9(thetaL)
  thetaM/1 -> ANDI Inversion/10(thetaM)
  thetaN/1 -> ANDI Inversion/11(thetaN)
  ANDI Inversion/1(u_model) -> u_ANDI/1
  Mux1/1 -> refs/1  "p_ref,q_ref,r_ref"
  ANDI Inversion/2(valid_B) -> valid_B/1
  Constant/1 -> Sum7/2
  Sum7/1 -> Gain1/1  "de trim ref."
  Constant1/1 -> Sum8/2
  Sum8/1 -> Gain/1  "da trim ref."
  Constant2/1 -> Sum9/2
  Sum9/1 -> Gain2/1  "dr trim ref."
  ANDI Inversion/3(nu_aw) -> Demux1/1
  Demux1/1 -> Gain10/1  "delta_nu_p"
  Demux1/2 -> Gain11/1  "delta_nu_q"
  Demux1/3 -> Gain12/1  "delta_nu_r"
  Gain5/1 -> Sum10/1
  Gain10/1 -> Sum10/2
  Sum10/1 -> Integrator/1
  Gain11/1 -> Sum11/2
  Sum12/1 -> Integrator2/1
  Gain12/1 -> Sum12/2

== system Citation_FlightGear_v2/Cessna Citation 500 ==
  note: p
      | q
      | r
      | vtas
      | alpha
      | beta
      | phi
      | theta
      | psi
      | he
      | xe
      | ye
  note: de
      | da
      | dr
      | dte
      | dta
      | dtr
      | df
      | gear
      | pla1
      | pla2
  note: pdot
      | qdot
      | rdot
      | VTASdot
      | hedot
  note: hradio
      | Mach
      | u_wind_e
      | v_wind_e
      | w_wind_e
  note: anxb
      | anyb
      | anzb
      | n
  note: gamma
      | chi
      | Vground
  note: turb 8x
      | terr_elev
  note: flaps
      | gear
  note: de
      | da
      | dr
      | dte
      | dta
      | dtr
      | df
      | gear
      | pla1
      | pla2
  note: FFl
      | N1l
      | N2l
      | FFr
      | N1r
      | N2r
  Inputs : Inport
  Environment : Inport  Port=2
  Actuators : Subsystem
  Citation model DASMAT : Subsystem
  Controllers : Subsystem
  Demux4 : Demux  Outputs=[8 2]
      settings: DisplayOption=none
  Mux1 : Mux  Inputs=7
  Mux2 : Mux  Inputs=2
  trim conditions : Subsystem
  ua sel : Selector  IndexOptions=Index vector (dialog)  Indices=[5 6]  OutputSizes=1
  xdot sel : Selector  IndexOptions=Index vector (dialog)  Indices=[1 2 3 4 10]  OutputSizes=1
  yacc sel : Selector  IndexOptions=Index vector (dialog)  Indices=[4 5 6 15]  OutputSizes=1
  yair sel : Selector  IndexOptions=Index vector (dialog)  Indices=[6 9 22 23 24]  OutputSizes=1
  yfp sel : Selector  IndexOptions=Index vector (dialog)  Indices=[1 2 15]  OutputSizes=1
  ypp sel : Selector  IndexOptions=Index vector (dialog)  Indices=[2 3 4 13 14 15]  OutputSizes=1
  output : Outport
  Trimmed input : Outport  Port=2
  Outport SysID Deflections : Outport  Port=3
  wires:
  Mux1/1 -> output/1
  Citation model DASMAT/1(x) -> Mux1/1, Controllers/1(state)
  Inputs/1 -> Controllers/2(inputs)
  Demux4/1 -> Citation model DASMAT/1(ua), ua sel/1
  Demux4/2 -> Citation model DASMAT/2(ut)
  Environment/1 -> Citation model DASMAT/3(Environment)
  Citation model DASMAT/3(yair) -> yair sel/1
  yair sel/1 -> Mux1/3
  Citation model DASMAT/2(xdot) -> xdot sel/1
  xdot sel/1 -> Mux1/2
  yacc sel/1 -> Mux1/4
  Citation model DASMAT/4(yacc) -> yacc sel/1
  yfp sel/1 -> Mux1/5
  Citation model DASMAT/5(yfp) -> yfp sel/1
  Actuators/1(Out) -> Demux4/1
  trim conditions/1(ua) -> Mux2/1
  trim conditions/2(ut) -> Mux2/2
  Mux2/1 -> Trimmed input/1
  Controllers/1(control inputs) -> Actuators/1(In)
  ua sel/1 -> Mux1/7
  Citation model DASMAT/6(ypp) -> ypp sel/1
  ypp sel/1 -> Mux1/6
  Actuators/2(Outport SysID Deflections) -> Outport SysID Deflections/1

== system Citation_FlightGear_v2/Classical Rate Controller ==
  refs : Inport
  pqr : Inport  Port=2
  PI_reset : Inport  Port=3
  Constant : Constant  Value=u0(2)
  Constant1 : Constant  Value=u0(1)
  Constant2 : Constant  Value=u0(3)
  Demux : Demux  Outputs=3
  Demux1 : Demux  Outputs=3
  Gain : Gain  Gain=Kp_p_classical
  Gain1 : Gain  Gain=Ki_p_classical
  Gain2 : Gain  Gain=Kp_q_classical
  Gain3 : Gain  Gain=Ki_q_classical
  Gain4 : Gain  Gain=Kp_r_classical
  Gain5 : Gain  Gain=Ki_r_classical
  Integrator : Integrator  ExternalReset=rising
  Integrator1 : Integrator  ExternalReset=rising
  Integrator2 : Integrator  ExternalReset=rising
  Mux : Mux  Inputs=3
  Sum : Sum  Inputs=|+-
  Sum{1,3..5,7..8} (6 alike) : Sum  Inputs=|++
  Sum2 : Sum  Inputs=|+-
  Sum6 : Sum  Inputs=|+-
  To Workspace : ToWorkspace  VariableName=da_classical  SaveFormat=Timeseries  SampleTime=-1
  To Workspace1 : ToWorkspace  VariableName=dr_classical  SaveFormat=Timeseries  SampleTime=-1
  To Workspace2 : ToWorkspace  VariableName=de_classical  SaveFormat=Timeseries  SampleTime=-1
  u_classical : Outport
  wires:
  refs/1 -> Demux/1
  Demux/1 -> Sum/1  "p_ref"
  Demux/2 -> Sum2/1  "q_ref"
  Demux/3 -> Sum6/1  "r_ref"
  pqr/1 -> Demux1/1
  Demux1/1 -> Sum/2  "p"
  Demux1/3 -> Sum6/2  "r"
  Sum/1 -> Gain1/1, Gain/1  "e_p"
  Gain1/1 -> Integrator/1
  Gain/1 -> Sum1/1
  Integrator/1 -> Sum1/2
  Sum1/1 -> Sum4/1
  Demux1/2 -> Sum2/2  "q"
  Sum2/1 -> Gain3/1, Gain2/1  "e_q"
  Gain2/1 -> Sum3/1
  Gain3/1 -> Integrator1/1
  Sum3/1 -> Sum5/1
  Integrator1/1 -> Sum3/2
  Constant/1 -> Sum4/2
  Sum4/1 -> Mux/2, To Workspace/1  "da_classical"
  Constant1/1 -> Sum5/2
  Sum5/1 -> To Workspace2/1, Mux/1  "de_classical"
  Sum6/1 -> Gain5/1, Gain4/1  "e_r"
  Integrator2/1 -> Sum7/2
  Gain5/1 -> Integrator2/1
  Sum7/1 -> Sum8/1
  Constant2/1 -> Sum8/2
  Gain4/1 -> Sum7/1
  Sum8/1 -> To Workspace1/1, Mux/3  "dr_classical"
  Mux/1 -> u_classical/1  "de,da,dr classical"
  PI_reset/1 -> Integrator2/2, Integrator1/2, Integrator/2

== system Citation_FlightGear_v2/Control Mode Selector ==
  u_ANDI : Inport
  pilot_u : Inport  Port=2
  ANDI_enable : Inport  Port=3
  u_classical : Inport  Port=4
  Mux : Mux  Inputs=2
  Reshape : Reshape
  Selector1 : Selector  InputPortWidth=10  IndexOptions=Index vector (dialog)  Indices=[4 5 6 7 8 9 10]  OutputSizes=1
  Switch : Switch  Criteria=u2 > Threshold  Threshold=0.5  SaturateOnIntegerOverflow=off  InputSameDT=off
  aircraft_u : Outport
  wires:
  u_ANDI/1 -> Switch/1
  pilot_u/1 -> Selector1/1
  Selector1/1 -> Mux/2  "u_remaining"
  ANDI_enable/1 -> Switch/2
  Switch/1 -> Mux/1
  Mux/1 -> Reshape/1  "aircraft_u"
  Reshape/1 -> aircraft_u/1
  u_classical/1 -> Switch/3

== system Citation_FlightGear_v2/FlightGear Visualisation ==
  "[p,q,r]" : Inport
  " [phi, theta, psi]" : Inport  Port=2
  "[he, xe, ye]" : Inport  Port=3
  u : Inport  Port=4
  Constant : Constant  Value=0
  Generate Run Script : aerolibfltsims/Generate Run Script  Architecture=Win64  dataFlow=Send  GeometryModelName=Yak-36  AirportId=KSFO  RunwayId=10L  InitialAltitude=7224  InitialHeading=113  OffsetDistance=4.72  OffsetAzimuth=0  InstallScenery=off  DisableShaders=off  OriginAddress=127.0.0.1  DestinationPort=5502  OriginPort=5505  LocalAddress=127.0.0.1  OutputFileName=runfg30.bat  FlightGearBaseDirectory=D:\Program Files\FlightGear3.0
  "P, Q, R" : Scope
      settings: ActiveDisplayYMinimum=-2.789820175659862  ActiveDisplayYMaximum=3.3807681055005783  DataLoggingVariableName=ScopeData2
  Send net_fdm Packet to FlightGear : aerolibfltsims/Send net_fdm Packet to FlightGear  DestinationIpAddress=127.0.0.1  DestinationPort=5502  LocalIpPort=-1  varLen=off  SampleTime=-1
  Subsystem : Subsystem
  Sum1 : Sum  Inputs=|++
  "h, posN,posE " : Scope
      settings: TimeSpan=10  ActiveDisplayYMinimum=-20000  ActiveDisplayYMaximum=10000  DataLoggingVariableName=ScopeData5
  "h, posN,posE, offsets" : Constant  Value=[0 -1000 2000]
  phi,theta,psi : Scope
      settings: ActiveDisplayYMinimum=-14.69567  ActiveDisplayYMaximum=1.72975  DataLoggingVariableName=ScopeData3
  wires:
  "h, posN,posE, offsets"/1 -> Sum1/2
  Sum1/1 -> "h, posN,posE "/1, Subsystem/3(Xe)
  Constant/1 -> Subsystem/4(href)
  u/1 -> Subsystem/5(u)
  Subsystem/1(FG Packet) -> Send net_fdm Packet to FlightGear/1
  "[he, xe, ye]"/1 -> Sum1/1
  "[p,q,r]"/1 -> "P, Q, R"/1, Subsystem/1(pqr)
  " [phi, theta, psi]"/1 -> phi,theta,psi/1, Subsystem/2(phi theta psi)

== system Citation_FlightGear_v2/Monitoring Fault Detection ==
  note: MA2 = moving average of the squared innovation
      | AUTOCORR = autocorrelation function
      | VARIANCE = spectral analysis
  innovations : Inport
  Monitoring Metrics : MATLAB Function  TreatAsAtomicUnit=on
  Zero-Order Hold : ZeroOrderHold  SampleTime=0.01
  MA2 : Outport
  AUTOCORR : Outport  Port=2
  VARIANCE : Outport  Port=3
  wires:
  innovations/1 -> Zero-Order Hold/1
  Zero-Order Hold/1 -> Monitoring Metrics/1(innovations)
  Monitoring Metrics/1(MA2) -> MA2/1
  Monitoring Metrics/2(AUTOCORR) -> AUTOCORR/1
  Monitoring Metrics/3(VARIANCE) -> VARIANCE/1

== system Citation_FlightGear_v2/Pilot ==
  note: de
      | da
      | dr
      | dte
      | dta
      | dtr
      | df
      | gear
      | pla1
      | pla2
      | turb 8x
      | terr elev
  Virtual Joystick (if you don't have a real one!) : Subsystem
  Input : Outport
  wires:
  Virtual Joystick (if you don't have a real one!)/1(Virtual joystick input) -> Input/1

== system Citation_FlightGear_v2/Cessna Citation 500/Actuators ==
  note: de
      | da
      | dr
      | dte
      | dta
      | dtr
      | df
      | gear
      | pla1
      | pla2
  note: de
      | da
      | dr
      | dte
      | dta
      | dtr
      | df
      | gear
      | pla1
      | pla2
  In : Inport
  Add : Sum
  Constant : Constant  Value=-0.28
  Demux : Demux  Outputs=10
      settings: DisplayOption=none
  Failure Activation : Step  Time=60  SampleTime=0
  Gain : Gain  Gain=0.5
  Mux : Mux  Inputs=10
  Mux1 : Mux  Inputs=3
  Switch : Switch  Criteria=u2 > Threshold  Threshold=0.5  SaturateOnIntegerOverflow=off  InputSameDT=off
  To Workspace : ToWorkspace  VariableName=failure_activation  SaveFormat=Timeseries  SampleTime=-1
      settings: Save2DSignal=2-D array (concatenate along first dimension)
  To Workspace1 : ToWorkspace  VariableName=da_actual  SaveFormat=Timeseries  SampleTime=-1
  da : Subsystem
  da limits : Saturate  UpperLimit=0.65  LowerLimit=-0.65
  de : Subsystem
  de limits : Saturate  UpperLimit=0.26  LowerLimit=-0.35
  dr : Subsystem
  dr limits : Saturate  UpperLimit=0.38  LowerLimit=-0.38
  flaps : Subsystem
  gear : Subsystem
  Out : Outport
  Outport SysID Deflections : Outport  Port=2
  wires:
  In/1 -> Demux/1
  Mux/1 -> Out/1
  Demux/1 -> de/1(In)
  Demux/2 -> da/1(In)
  Demux/3 -> dr/1(In)
  de/1(Out) -> de limits/1
  da/1(Out) -> da limits/1
  da limits/1 -> Mux1/2, Gain/1, Switch/3  "da_healthy"
  dr/1(Out) -> dr limits/1
  dr limits/1 -> Mux1/3, Mux/3  "dr_healthy"
  de limits/1 -> Mux1/1, Mux/1  "de_healthy"
  Demux/8 -> gear/1(In)
  Demux/7 -> flaps/1(In)
  Demux/9 -> Mux/9
  Demux/10 -> Mux/10
  flaps/1(Out) -> Mux/7
  gear/1(Out) -> Mux/8
  Demux/4 -> Mux/4
  Demux/5 -> Mux/5
  Demux/6 -> Mux/6
  Gain/1 -> Add/2
  Constant/1 -> Add/1
  Add/1 -> Switch/1  "da_failed"
  Switch/1 -> To Workspace1/1, Mux/2  "da_actual"
  Failure Activation/1 -> Switch/2, To Workspace/1
  Mux1/1 -> Outport SysID Deflections/1

== system Citation_FlightGear_v2/Cessna Citation 500/Citation model DASMAT ==
  ua : Inport
  ut : Inport  Port=2
  Environment : Inport  Port=3
  AIRCRAFT MODEL : Subsystem
  Mux1 : Mux  Inputs=[8 2 8 12 8]
  Terminator_{16..19} (4 alike) : Terminator
  massinit : Constant  Value=massinit
  x : Outport
  xdot : Outport  Port=2
  yair : Outport  Port=3
  yacc : Outport  Port=4
  yfp : Outport  Port=5
  ypp : Outport  Port=6
  wires:
  AIRCRAFT MODEL/13(FMt) -> Terminator_19/1
  Mux1/1 -> yair/1
  AIRCRAFT MODEL/12(FMag) -> Terminator_17/1
  AIRCRAFT MODEL/11(FMa) -> Terminator_18/1
  AIRCRAFT MODEL/7(gust) -> Mux1/5
  AIRCRAFT MODEL/6(wind) -> Mux1/4
  AIRCRAFT MODEL/5(yad2) -> Mux1/3
  AIRCRAFT MODEL/4(yad1) -> Mux1/2
  AIRCRAFT MODEL/3(yatm) -> Mux1/1
  AIRCRAFT MODEL/2(xdot) -> xdot/1
  AIRCRAFT MODEL/1(x) -> x/1
  AIRCRAFT MODEL/10(ys) -> Terminator_16/1
  AIRCRAFT MODEL/9(yfp) -> yfp/1
  AIRCRAFT MODEL/8(yacc) -> yacc/1
  ut/1 -> AIRCRAFT MODEL/2(ut)
  ua/1 -> AIRCRAFT MODEL/1(ua)
  Environment/1 -> AIRCRAFT MODEL/4(Environment)
  AIRCRAFT MODEL/14(ypp) -> ypp/1
  massinit/1 -> AIRCRAFT MODEL/3(massinit)

== system Citation_FlightGear_v2/Cessna Citation 500/Controllers ==
  state : Inport
  inputs : Inport  Port=2
  A/T disabled : Gain  Gain=0  SaturateOnIntegerOverflow=on  OutDataTypeStr=Inherit: Same as input  ParamDataTypeStr=Inherit: Same as input
  Yaw damper : Subsystem
  add controller outputs to pilot inputs : Sum  Inputs=|+|+|+|  SaturateOnIntegerOverflow=on
  auto throttle : Subsystem
  control inputs : Outport
  wires:
  state/1 -> Yaw damper/1(state), auto throttle/1(state)
  inputs/1 -> Yaw damper/2(inputs), add controller outputs to pilot inputs/3, auto throttle/2(inputs)
  add controller outputs to pilot inputs/1 -> control inputs/1
  Yaw damper/1(controller output) -> add controller outputs to pilot inputs/1
  auto throttle/1(controller output) -> A/T disabled/1
  A/T disabled/1 -> add controller outputs to pilot inputs/2

== system Citation_FlightGear_v2/Cessna Citation 500/trim conditions ==
  PLA1/Tx1 : Constant  Value=ut0(1)
  PLA2/Tx2 : Constant  Value=ut0(2)
  control inputs : Mux  Inputs=8
      settings: DisplayOption=signals
  deltaa : Constant  Value=u0(2)
  deltae : Constant  Value=u0(1)
  deltaf : Constant  Value=u0(7)
  deltar : Constant  Value=u0(3)
  deltata : Constant  Value=u0(5)
  deltate : Constant  Value=u0(4)
  deltatr : Constant  Value=u0(6)
  engine inputs : Mux  Inputs=2
      settings: DisplayOption=signals
  lgsw : Constant  Value=u0(8)
  ua : Outport
  ut : Outport  Port=2
  wires:
  deltaf/1 -> control inputs/7  "df"
  engine inputs/1 -> ut/1
  deltatr/1 -> control inputs/6  "dtr"
  deltata/1 -> control inputs/5  "dta"
  control inputs/1 -> ua/1
  PLA1/Tx1/1 -> engine inputs/1  "pla1"
  PLA2/Tx2/1 -> engine inputs/2  "pla2"
  deltae/1 -> control inputs/1  "de"
  deltaa/1 -> control inputs/2  "da"
  deltar/1 -> control inputs/3  "dr"
  deltate/1 -> control inputs/4  "dte"
  lgsw/1 -> control inputs/8  "lg"

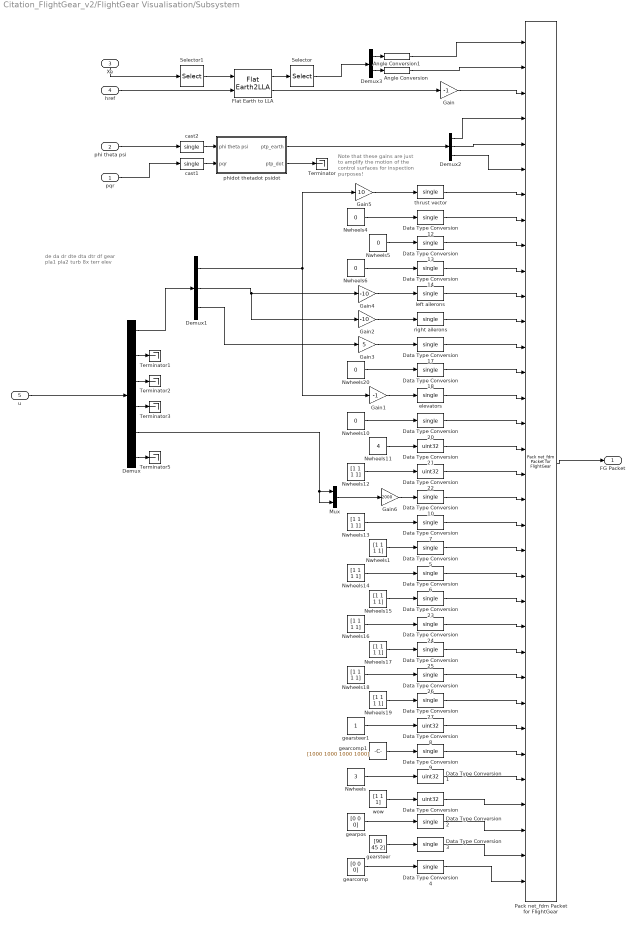
== system Citation_FlightGear_v2/FlightGear Visualisation/Subsystem ==
  note: Note that these gains are just to amplify the motion of the control surfaces for inspection purposes!
  note: de
      | da
      | dr
      | dte
      | dta
      | dtr
      | df
      | gear
      | pla1
      | pla2
      | turb 8x
      | terr elev
  pqr : Inport
  phi theta psi : Inport  Port=2
  Xe : Inport  Port=3
  href : Inport  Port=4
  u : Inport  Port=5
  Angle Conversion : aerolibconvert2/Angle Conversion  IU=deg  OU=rad
  Angle Conversion1 : aerolibconvert2/Angle Conversion  IU=deg  OU=rad
  Data Type Conversion{,1,8,21..22} (5 alike) : DataTypeConversion  OutDataTypeStr=uint32  SaturateOnIntegerOverflow=off  RndMeth=Floor
  Data Type Conversion{2..7,9..10,12..14,17..18,20,23..27} (19 alike) : DataTypeConversion  OutDataTypeStr=single  SaturateOnIntegerOverflow=off  RndMeth=Floor
  Demux : Demux  Outputs=[3 3 1 1 2 9]
  Demux1 : Demux  Outputs=[1 1 1]
  Demux2 : Demux  Outputs=3
  Demux3 : Demux  Outputs=2
  Flat Earth to LLA : FlatEarth2LLA  R=6378137  LL0=[37.7889 -122.4778]
  Gain : Gain  Gain=-1
  Gain1 : Gain  Gain=-1
  Gain2 : Gain  Gain=-10
  Gain3 : Gain  Gain=5
  Gain4 : Gain  Gain=-10
  Gain5 : Gain  Gain=10
  Gain6 : Gain  Gain=2000
  Mux : Mux  Inputs=2
  Nwheels : Constant  Value=3
  Nwheels{1,12..19} (9 alike) : Constant  Value=[1 1 1 1]
  Nwheels{4..6,10,20} (5 alike) : Constant  Value=0
  Nwheels11 : Constant  Value=4
  Pack net_fdm Packet for FlightGear : aerolibfltsims/Pack net_fdm Packet for FlightGear  FlightGearVersion=v2016.1  ShowPositionAttitudeInputs=on  ShowVelocityAccelerationInputs=off  ShowControlSurfacePositionInputs=on  ShowEngineFuelInputs=on  ShowLandingGearInputs=on  ShowEnvironmentInputs=off  SampleTime=-1  packetVersion=24
  Selector : Selector  InputPortWidth=2  IndexOptions=Index vector (dialog)  Indices=[2 1]  OutputSizes=1
  Selector1 : Selector  InputPortWidth=3  IndexOptions=Index vector (dialog)  Indices=[2 3 1]  OutputSizes=1
  Terminator{,1..3,5} (5 alike) : Terminator
  cast1 : DataTypeConversion  OutDataTypeStr=single  RndMeth=Floor
  cast2 : DataTypeConversion  OutDataTypeStr=single  RndMeth=Floor
  elevators : DataTypeConversion  OutDataTypeStr=single  SaturateOnIntegerOverflow=off  RndMeth=Floor
  gearcomp : Constant  Value=[0 0 0]
  gearcomp1 : Constant  Value=[1000 1000 1000 1000]
  gearpos : Constant  Value=[0 0 0]  VectorParams1D=off
  gearsteer : Constant  Value=[90 45 2]
  gearsteer1 : Constant
  left ailerons : DataTypeConversion  OutDataTypeStr=single  SaturateOnIntegerOverflow=off  RndMeth=Floor
  phidot thetadot psidot : Subsystem
  right ailerons : DataTypeConversion  OutDataTypeStr=single  SaturateOnIntegerOverflow=off  RndMeth=Floor
  thrust vector : DataTypeConversion  OutDataTypeStr=single  SaturateOnIntegerOverflow=off  RndMeth=Floor
  wow : Constant  Value=[1 1 1]
  FG Packet : Outport  VectorParamsAs1DForOutWhenUnconnected=off
  wires:
  Pack net_fdm Packet for FlightGear/1 -> FG Packet/1
  href/1 -> Flat Earth to LLA/2
  Flat Earth to LLA/1 -> Selector/1
  Selector/1 -> Demux3/1
  Demux3/1 -> Angle Conversion1/1
  Demux3/2 -> Angle Conversion/1
  Angle Conversion1/1 -> Pack net_fdm Packet for FlightGear/1
  phidot thetadot psidot/1(ptp_earth) -> Demux2/1
  Demux2/1 -> Pack net_fdm Packet for FlightGear/4
  Demux2/2 -> Pack net_fdm Packet for FlightGear/5
  Demux2/3 -> Pack net_fdm Packet for FlightGear/6
  phidot thetadot psidot/2(ptp_dot) -> Terminator/1
  pqr/1 -> cast1/1
  Angle Conversion/1 -> Pack net_fdm Packet for FlightGear/2
  Flat Earth to LLA/2 -> Gain/1
  Gain/1 -> Pack net_fdm Packet for FlightGear/3
  Data Type Conversion17/1 -> Pack net_fdm Packet for FlightGear/13
  Data Type Conversion8/1 -> Pack net_fdm Packet for FlightGear/28
  Nwheels13/1 -> Data Type Conversion7/1
  Data Type Conversion25/1 -> Pack net_fdm Packet for FlightGear/25
  left ailerons/1 -> Pack net_fdm Packet for FlightGear/11
  Nwheels15/1 -> Data Type Conversion23/1
  Nwheels19/1 -> Data Type Conversion27/1
  Data Type Conversion12/1 -> Pack net_fdm Packet for FlightGear/8
  Data Type Conversion9/1 -> Pack net_fdm Packet for FlightGear/29
  Demux1/2 -> Gain2/1, Gain4/1
  Data Type Conversion21/1 -> Pack net_fdm Packet for FlightGear/17
  Data Type Conversion14/1 -> Pack net_fdm Packet for FlightGear/10
  Data Type Conversion6/1 -> Pack net_fdm Packet for FlightGear/22
  thrust vector/1 -> Pack net_fdm Packet for FlightGear/7
  Nwheels6/1 -> Data Type Conversion14/1
  Nwheels12/1 -> Data Type Conversion22/1
  Nwheels14/1 -> Data Type Conversion6/1
  Nwheels5/1 -> Data Type Conversion13/1
  right ailerons/1 -> Pack net_fdm Packet for FlightGear/12
  Data Type Conversion22/1 -> Pack net_fdm Packet for FlightGear/18
  gearcomp1/1 -> Data Type Conversion9/1
  Data Type Conversion13/1 -> Pack net_fdm Packet for FlightGear/9
  Data Type Conversion26/1 -> Pack net_fdm Packet for FlightGear/26
  Nwheels1/1 -> Data Type Conversion5/1
  gearsteer1/1 -> Data Type Conversion8/1
  elevators/1 -> Pack net_fdm Packet for FlightGear/15
  Data Type Conversion18/1 -> Pack net_fdm Packet for FlightGear/14
  Data Type Conversion20/1 -> Pack net_fdm Packet for FlightGear/16
  Nwheels10/1 -> Data Type Conversion20/1
  Xe/1 -> Selector1/1
  Data Type Conversion10/1 -> Pack net_fdm Packet for FlightGear/19
  Nwheels4/1 -> Data Type Conversion12/1
  Data Type Conversion27/1 -> Pack net_fdm Packet for FlightGear/27
  Data Type Conversion4/1 -> Pack net_fdm Packet for FlightGear/34
  gearpos/1 -> Data Type Conversion2/1
  Data Type Conversion2/1 -> Pack net_fdm Packet for FlightGear/32
  Data Type Conversion3/1 -> Pack net_fdm Packet for FlightGear/33
  Nwheels/1 -> Data Type Conversion1/1
  wow/1 -> Data Type Conversion/1
  gearsteer/1 -> Data Type Conversion3/1
  Data Type Conversion1/1 -> Pack net_fdm Packet for FlightGear/30
  gearcomp/1 -> Data Type Conversion4/1
  Data Type Conversion/1 -> Pack net_fdm Packet for FlightGear/31
  Nwheels17/1 -> Data Type Conversion25/1
  Nwheels16/1 -> Data Type Conversion24/1
  Data Type Conversion23/1 -> Pack net_fdm Packet for FlightGear/23
  Data Type Conversion24/1 -> Pack net_fdm Packet for FlightGear/24
  Nwheels11/1 -> Data Type Conversion21/1
  Data Type Conversion7/1 -> Pack net_fdm Packet for FlightGear/20
  Data Type Conversion5/1 -> Pack net_fdm Packet for FlightGear/21
  Nwheels18/1 -> Data Type Conversion26/1
  cast2/1 -> phidot thetadot psidot/1(phi theta psi)
  cast1/1 -> phidot thetadot psidot/2(pqr)
  phi theta psi/1 -> cast2/1
  Demux1/3 -> Gain3/1
  Nwheels20/1 -> Data Type Conversion18/1
  u/1 -> Demux/1
  Gain1/1 -> elevators/1
  Demux1/1 -> Gain1/1, Gain5/1
  Demux/1 -> Demux1/1
  Gain2/1 -> right ailerons/1
  Demux/2 -> Terminator1/1
  Demux/3 -> Terminator2/1
  Demux/4 -> Terminator3/1
  Demux/6 -> Terminator5/1
  Selector1/1 -> Flat Earth to LLA/1
  Gain3/1 -> Data Type Conversion17/1
  Gain4/1 -> left ailerons/1
  Gain5/1 -> thrust vector/1
  Demux/5 -> Mux/1, Mux/2
  Mux/1 -> Gain6/1
  Gain6/1 -> Data Type Conversion10/1
